simulink model "Rotary_Parking_System_state_flow"  (R2019a)
settings: Solver=VariableStepAuto  StartTime=0.0  StopTime=inf  RelTol=1e-3
settings Model: Creator=mmb94  LastModifiedBy=mmb94

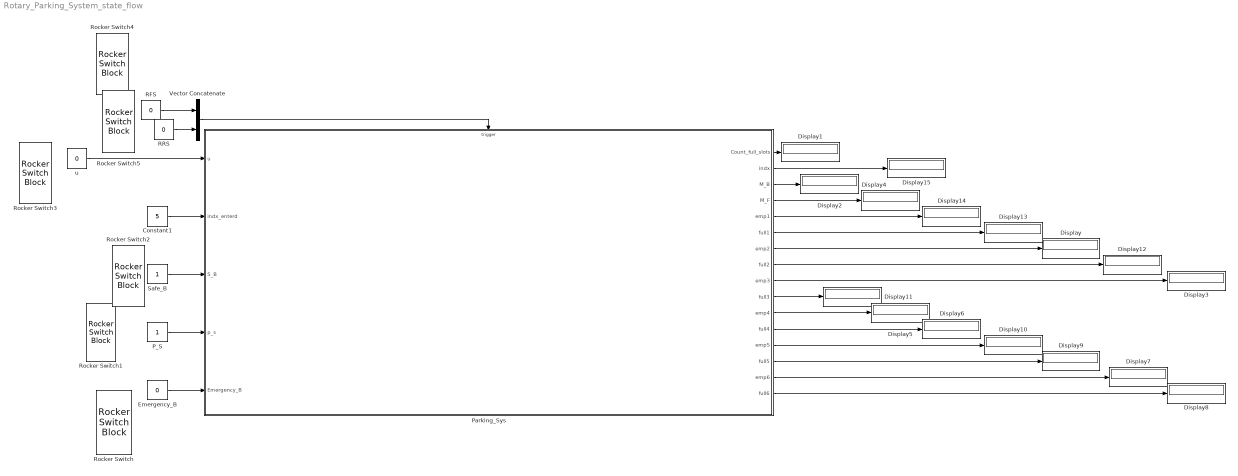
== system Rotary_Parking_System_state_flow ==
  Constant1 : Constant  Value=5
  Display{,1..15} (16 alike) : Display
  Emergency_B : Constant  Value=0
  P_S : Constant
  Parking_Sys : Stateflow chart  BlockKeywords=__PRM__SERIALIZED__DATA__:Stateflow Chart,Stateflow Diagram  TreatAsAtomicUnit=on
  RFS : Constant  Value=0
  RRS : Constant  Value=0
  Rocker Switch{,1..5} (6 alike) : RockerSwitchBlock
      settings: Values={{'Off', 'On'}, [0 1]}
  Safe_B : Constant
  Vector Concatenate : Concatenate
  u : Constant  Value=0
  wires:
  Parking_Sys/1(Count_full_slots) -> Display1/1
  Parking_Sys/9(emp3) -> Display3/1
  Parking_Sys/4(M_F) -> Display4/1
  Parking_Sys/12(full4) -> Display6/1
  Parking_Sys/14(full5) -> Display9/1
  Parking_Sys/16(full6) -> Display8/1
  Parking_Sys/15(emp6) -> Display7/1
  Parking_Sys/13(emp5) -> Display10/1
  Parking_Sys/11(emp4) -> Display5/1
  Parking_Sys/10(full3) -> Display11/1
  Parking_Sys/8(full2) -> Display12/1
  Parking_Sys/7(emp2) -> Display/1
  Parking_Sys/6(full1) -> Display13/1
  Parking_Sys/5(emp1) -> Display14/1
  Parking_Sys/3(M_B) -> Display2/1
  Vector Concatenate/1 -> Parking_Sys/Trigger
  RFS/1 -> Vector Concatenate/1
  u/1 -> Parking_Sys/1(u)
  Constant1/1 -> Parking_Sys/2(indx_enterd)
  Safe_B/1 -> Parking_Sys/3(S_B)
  P_S/1 -> Parking_Sys/4(p_s)
  Emergency_B/1 -> Parking_Sys/5(Emergency_B)
  RRS/1 -> Vector Concatenate/2
  Parking_Sys/2(indx) -> Display15/1

== stateflow chart Rotary_Parking_System_state_flow/Parking_Sys ==
  state System
    state Power_on
      state Slots [parallel]
        entry: emp1 = 1;
        entry:emp2 = 1;
        entry:emp3 = 1;
        entry:emp4 = 1;
        entry:emp5 = 1;
        entry:emp6 = 1;
        entry: full1 = 0;
        entry: full2=0;
        entry: full3=0;
        entry: full4=0;
        entry: full5=0;
        entry: full6=0;
        settings: executionOrder=1
        state Slot1
          entry: indx =1;
          entry: M_F=0;
          entry: M_B=0;
          state check
          state Full
            entry: full1 = 1;
          state Empty
            entry: emp1 = 1;
          (default) -> System.Power_on.Slots.Slot1.check
          System.Power_on.Slots.Slot1.check -> System.Power_on.Slots.Slot1.Full [order 2] : [full1==1&&emp1==0]
          System.Power_on.Slots.Slot1.check -> System.Power_on.Slots.Slot1.Empty [order 1] : [emp1==1&& full1==0]
          System.Power_on.Slots.Slot1.Empty -> System.Power_on.Slots.Slot1.Full [order 1] : R_F_S[u == 0]{emp1=0;}
          System.Power_on.Slots.Slot1.Full -> System.Power_on.Slots.Slot1.Empty [order 1] : R_R_S[indx_enterd == indx && u==1]{full1=0;}
        state Slot6
          entry: indx =6;
          entry: M_F=0;
          entry: M_B=0;
          state check
          state Full
            entry: full6 = 1;
          state Empty
            entry: emp6 = 1;
          (default) -> System.Power_on.Slots.Slot6.check
          System.Power_on.Slots.Slot6.check -> System.Power_on.Slots.Slot6.Empty [order 2] : [emp6==1&& full6==0]
          System.Power_on.Slots.Slot6.check -> System.Power_on.Slots.Slot6.Full [order 1] : [full6==1&&emp6==0]
          System.Power_on.Slots.Slot6.Empty -> System.Power_on.Slots.Slot6.Full [order 1] : R_F_S[u == 0]{emp6=0;}
          System.Power_on.Slots.Slot6.Full -> System.Power_on.Slots.Slot6.Empty [order 3] : R_R_S[indx_enterd == indx && u==1]{full6=0;}
        state Slot2
          entry: indx =2;
          entry: M_F=0;
          entry: M_B=0;
          state check
          state Empty
            entry: emp2 = 1;
          state Full
            entry: full2 = 1;
          (default) -> System.Power_on.Slots.Slot2.check
          System.Power_on.Slots.Slot2.check -> System.Power_on.Slots.Slot2.Full [order 2] : [full2==1&&emp2==0]
          System.Power_on.Slots.Slot2.check -> System.Power_on.Slots.Slot2.Empty [order 1] : [emp2==1&& full2==0]
          System.Power_on.Slots.Slot2.Empty -> System.Power_on.Slots.Slot2.Full [order 1] : R_F_S[u==0]{emp2=0;}
          System.Power_on.Slots.Slot2.Full -> System.Power_on.Slots.Slot2.Empty [order 3] : R_R_S[indx_enterd==indx && u==1]{full2=0;}
        state Slot5
          entry: indx=5;
          entry: M_F=0;
          entry: M_B=0;
          state check
          state Empty
            entry: emp5 = 1;
          state Full
            entry: full5 = 1;
          (default) -> System.Power_on.Slots.Slot5.check
          System.Power_on.Slots.Slot5.check -> System.Power_on.Slots.Slot5.Full [order 2] : [full5==1&&emp5==0]
          System.Power_on.Slots.Slot5.check -> System.Power_on.Slots.Slot5.Empty [order 1] : [emp4==1&& full4==0]
          System.Power_on.Slots.Slot5.Empty -> System.Power_on.Slots.Slot5.Full [order 2] : R_F_S[u == 0]{emp5=0;}
          System.Power_on.Slots.Slot5.Full -> System.Power_on.Slots.Slot5.Empty [order 1] : R_R_S[indx_enterd == indx && u==1]{full5=0;}
        state Slot4
          entry: indx =4;
          entry: M_F=0;
          entry: M_B=0;
          state check
          state Empty
            entry: emp4 = 1;
          state Full
            entry: full4 = 1;
          (default) -> System.Power_on.Slots.Slot4.check
          System.Power_on.Slots.Slot4.check -> System.Power_on.Slots.Slot4.Empty [order 1] : [emp4==1&& full4==0]
          System.Power_on.Slots.Slot4.check -> System.Power_on.Slots.Slot4.Full [order 2] : [full4==1&&emp4==0]
          System.Power_on.Slots.Slot4.Empty -> System.Power_on.Slots.Slot4.Full [order 1] : R_F_S[u==0]{emp4=0;}
          System.Power_on.Slots.Slot4.Full -> System.Power_on.Slots.Slot4.Empty [order 1] : R_R_S[indx_enterd==indx && u==1]{full4=0;}
        state Slot3
          entry: indx =3;
          entry: M_F=0;
          entry: M_B=0;
          state check
          state Full
            entry: full3 = 1;
          state Empty
            entry: emp3 = 1;
          (default) -> System.Power_on.Slots.Slot3.check
          System.Power_on.Slots.Slot3.check -> System.Power_on.Slots.Slot3.Full [order 1] : [full3==1&&emp3==0]
          System.Power_on.Slots.Slot3.check -> System.Power_on.Slots.Slot3.Empty [order 2] : [emp3==1&& full3==0]
          System.Power_on.Slots.Slot3.Full -> System.Power_on.Slots.Slot3.Empty [order 1] : R_R_S[indx_enterd==indx && u==1]{full3=0;}
          System.Power_on.Slots.Slot3.Empty -> System.Power_on.Slots.Slot3.Full [order 1] : R_F_S[u==0]{emp3=0;}
        (default) -> Slot1
        System.Power_on.Slots.Slot1.Empty -> Slot6 [order 3] : R_R_S[indx_enterd ~= indx && (indx_enterd>3) ]{M_B=1}
        System.Power_on.Slots.Slot6.Empty -> Slot1 [order 3] : R_R_S[indx_enterd ~= indx && (3<indx_enterd<indx) ]{M_B=1}
        System.Power_on.Slots.Slot1.Full -> Slot6 [order 4] : R_F_S[(emp6==1 | emp5==1)&&( full2==1)&& S_B==1]{M_B=1}
        System.Power_on.Slots.Slot1.Full -> Slot6 [order 5] : R_R_S[indx_enterd ~= indx && (indx_enterd>3) ]{M_B=1}
        System.Power_on.Slots.Slot1.Full -> Slot2 [order 3] : R_F_S[(emp2==1 | emp3==1 | emp4==1) && S_B==1]{M_F=1}
        System.Power_on.Slots.Slot1.Full -> Slot2 [order 2] : R_R_S[(indx_enterd ~=indx) && (indx<indx_enterd<=3) ]{M_F=1}
        System.Power_on.Slots.Slot1.Empty -> Slot2 [order 2] : R_R_S[(indx_enterd ~=indx) && (indx<indx_enterd<=3) ]{M_F=1}
        System.Power_on.Slots.Slot6.Full -> Slot1 [order 1] : R_F_S[( emp1==1 | emp2==1 | emp3==1 )&& ( full5==1 )&& S_B ==1]{M_B=1}
        System.Power_on.Slots.Slot6.Full -> Slot1 [order 2] : R_R_S[indx_enterd ~= indx && (3<indx_enterd<indx) ]{M_B=1}
        System.Power_on.Slots.Slot2.Empty -> Slot1 [order 2] : R_R_S[indx_enterd ~= indx && (indx_enterd<indx | indx_enterd>4) ]{M_B=1}
        System.Power_on.Slots.Slot2.Full -> Slot1 [order 1] : R_F_S[(emp1==1 | emp6==1)&&( full3==1) && S_B ==1]{M_B=1}
        System.Power_on.Slots.Slot2.Full -> Slot1 [order 2] : R_R_S[indx_enterd ~= indx && (indx_enterd<indx | indx_enterd>4) ]{M_B=1}
        System.Power_on.Slots.Slot6.Full -> Slot5 [order 4] : R_F_S[(emp4==1 | emp5==1)&&( full1==1) && S_B ==1]{M_B=1}
        System.Power_on.Slots.Slot6.Full -> Slot5 [order 5] : R_R_S[indx_enterd ~= indx && (indx_enterd<indx ) ]{M_B=1}
        System.Power_on.Slots.Slot6.Empty -> Slot5 [order 2] : R_R_S[indx_enterd ~= indx && (indx_enterd<indx ) ]{M_B=1}
        System.Power_on.Slots.Slot5.Full -> Slot6 [order 5] : R_R_S[(indx_enterd ~=indx) &&( (indx<indx_enterd)| indx_enterd<3 )]{M_F=1}
        System.Power_on.Slots.Slot5.Full -> Slot6 [order 4] : R_F_S[( emp6==1 | emp1==1 | emp2==1 )&&( full4==1 ) && S_B==1]{M_F=1}
        System.Power_on.Slots.Slot5.Empty -> Slot6 [order 3] : R_R_S[(indx_enterd ~=indx) &&( (indx<indx_enterd)| indx_enterd<3 )]{M_F=1}
        System.Power_on.Slots.Slot2.Empty -> Slot3 [order 3] : R_R_S[(indx_enterd ~=indx) && (indx<indx_enterd<=3)]{M_F=1}
        System.Power_on.Slots.Slot2.Full -> Slot3 [order 4] : R_F_S[( emp3==1 | emp4==1 | emp5==1 )&&( full1==1) && S_B==1]{M_F=1}
        System.Power_on.Slots.Slot2.Full -> Slot3 [order 5] : R_R_S[(indx_enterd ~=indx) && (indx<indx_enterd<=3)]{M_F=1}
        System.Power_on.Slots.Slot3.Empty -> Slot2 [order 2] : R_R_S[indx_enterd ~= indx && (indx_enterd<indx ) ]{M_B=1}
        System.Power_on.Slots.Slot3.Full -> Slot2 [order 2] : R_F_S[(emp1==1 | emp2==1)&&( full4==1)&& S_B ==1]{M_B=1}
        System.Power_on.Slots.Slot3.Full -> Slot2 [order 3] : R_R_S[indx_enterd ~= indx && (indx_enterd<indx ) ]{M_B=1}
        System.Power_on.Slots.Slot5.Full -> Slot4 [order 2] : R_F_S[(emp3==1 | emp4==1)&& (full6==1) && S_B ==1]{M_B=1}
        System.Power_on.Slots.Slot5.Full -> Slot4 [order 3] : R_R_S[indx_enterd ~= indx && (indx_enterd<indx ) ]{M_B=1}
        System.Power_on.Slots.Slot5.Empty -> Slot4 [order 1] : R_R_S[indx_enterd ~= indx && (indx_enterd<indx ) ]{M_B=1}
        System.Power_on.Slots.Slot4.Full -> Slot5 [order 5] : R_F_S[( emp5==1 | emp6==1| emp1==1 )&&( full3==1 ) && S_B==1]{M_F=1}
        System.Power_on.Slots.Slot4.Full -> Slot5 [order 4] : R_R_S[(indx_enterd ~=indx) && (indx<indx_enterd)]{M_F=1}
        System.Power_on.Slots.Slot4.Empty -> Slot5 [order 3] : R_R_S[(indx_enterd ~=indx) && (indx<indx_enterd)]{M_F=1}
        System.Power_on.Slots.Slot3.Empty -> Slot4 [order 3] : R_R_S[(indx_enterd ~=indx) && (indx<indx_enterd)]{M_F=1}
        System.Power_on.Slots.Slot4.Empty -> Slot3 [order 2] : R_R_S[indx_enterd ~= indx && (indx_enterd<indx ) ]{M_B=1}
        System.Power_on.Slots.Slot3.Full -> Slot4 [order 4] : R_F_S[(emp4==1 | emp5==1 | emp6==1)&&( full2==1 ) && S_B==1]{M_F=1}
        System.Power_on.Slots.Slot3.Full -> Slot4 [order 5] : R_R_S[(indx_enterd ~=indx) && (indx<indx_enterd)]{M_F=1}
        System.Power_on.Slots.Slot4.Full -> Slot3 [order 2] : R_F_S[(emp2==1 | emp3==1 )&&( full5==1)& S_B ==1]{M_B=1}
        System.Power_on.Slots.Slot4.Full -> Slot3 [order 3] : R_R_S[indx_enterd ~= indx && (indx_enterd<indx ) ]{M_B=1}
      state LCD [parallel]
        settings: executionOrder=2
        state Count_full_slot [parallel]
          during: Count_full_slots = full1+ full2 +full3+full4+full5+full6
          settings: executionOrder=1
    state Power_off1
      entry: M_F=0;
      entry: M_B=0;
    Power_off1 -> Power_on : [p_s ==1]
    Power_on -> Power_off1 : [p_s ==0]
    (default) -> Power_off1
  state Emergency_stop
    entry: M_F=0;
    entry: M_B=0;
    entry: Count_full_slots =-1;
  (default) -> System
  Emergency_stop -> System : [Emergency_B==0]
  System -> Emergency_stop : [Emergency_B==1]
  data: u input; indx_enterd input; S_B input; p_s input; Count_full_slots output; indx output; M_B output; M_F output; emp1 output; full1 output; Emergency_B input; emp2 output; full2 output; emp3 output; full3 output; emp4 output; full4 output; emp5 output; full5 output; emp6 output; full6 output
  events: R_F_S input RISING_EDGE_EVENT; R_R_S input RISING_EDGE_EVENT
